simulink model "sliding_mode_controller"  (R2020a)
settings: Solver=ode1  StartTime=0.0  StopTime=50  FixedStep=0.01  RelTol=1e-3
model workspace (MAT data in the model file):
  kd = 0
  kp = 0
libraries: simulink x1, sharedutil x1
settings Model: Creator=Sebas  LastModifiedBy=Sebas
settings SolverCC: ConcurrentTasks=on  ZeroCrossAlgorithm=Adaptive  AlgebraicLoopSolver=LineSearch
settings DebuggingCC: MaskedZcDiagnostic=none  IgnoredZcDiagnostic=none

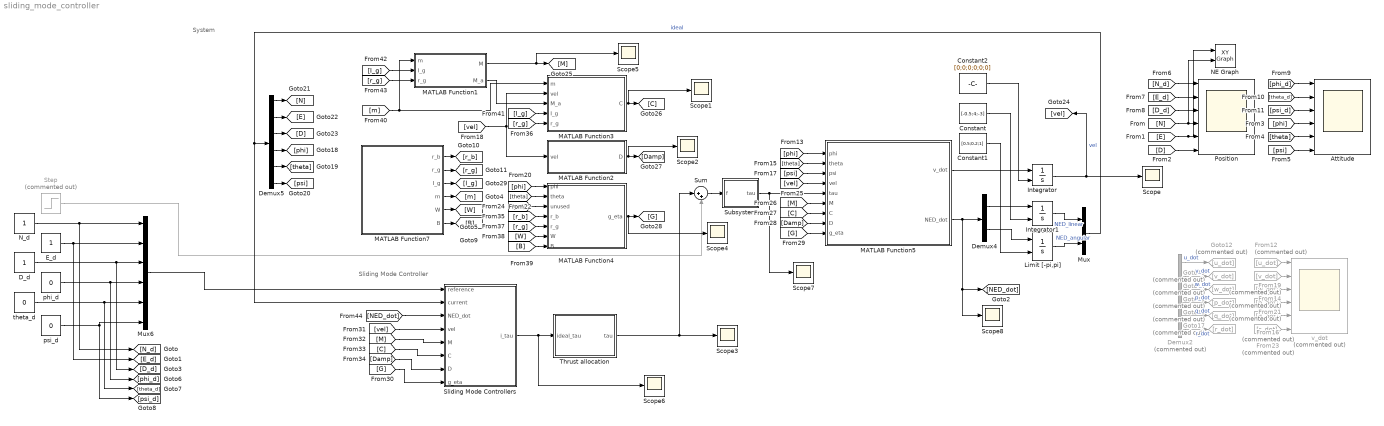
== system sliding_mode_controller ==
  note: System
  note: Sliding Mode Controller
  Attitude : Scope  NumInputPorts=6
  Constant : Constant  Value=[-0.5;4;-3]
  Constant1 : Constant  Value=[0.5;0.2;1]
  Constant2 : Constant  Value=[0;0;0;0;0;0]
  D_d : Constant
  Demux2 : Demux  Commented=on  Outputs=6
  Demux4 : Demux  Outputs=2
  Demux5 : Demux  Outputs=6
  E_d : Constant
  From12 : From  Commented=on  GotoTag=u_dot
  From14 : From  Commented=on  GotoTag=w_dot
  From16 : From  Commented=on  GotoTag=q_dot
  From19 : From  Commented=on  GotoTag=v_dot
  From21 : From  Commented=on  GotoTag=p_dot
  From23 : From  Commented=on  GotoTag=r_dot
  Goto12 : Goto  Commented=on  GotoTag=u_dot
  Goto13 : Goto  Commented=on  GotoTag=v_dot
  Goto14 : Goto  Commented=on  GotoTag=w_dot
  Goto15 : Goto  Commented=on  GotoTag=p_dot
  Goto16 : Goto  Commented=on  GotoTag=q_dot
  Goto17 : Goto  Commented=on  GotoTag=r_dot
  Integrator : Integrator  InitialConditionSource=external
  Integrator1 : Integrator  InitialConditionSource=external
  Limit [-pi,pi] : Integrator  InitialConditionSource=external  WrapState=on
  MATLAB Function1 : MATLAB Function  TreatAsAtomicUnit=on
  MATLAB Function2 : MATLAB Function  TreatAsAtomicUnit=on
  MATLAB Function3 : MATLAB Function  TreatAsAtomicUnit=on
  MATLAB Function4 : MATLAB Function  TreatAsAtomicUnit=on
  MATLAB Function5 : MATLAB Function  TreatAsAtomicUnit=on
  MATLAB Function7 : MATLAB Function  TreatAsAtomicUnit=on
  Mux : Mux  Inputs=2
  Mux6 : Mux  Inputs=6
  NE Graph : simulink/Sinks/XY Graph  xmin=-1  xmax=5  ymin=-1  ymax=2  st=-1
  N_d : Constant
  Position : Scope  NumInputPorts=6
  Scope{,1..8} (9 alike) : Scope
  Sliding Mode Controllers : Subsystem  mask(6 DOF Sliding Mode Controller){surge_k=3, sway_k=3, heave_k=4, roll_k=10, pitch_k=2, yaw_k=5, lambda=1, lambda_roll=5, lambda_pitch=3}
      mask prompts: surge_k "Surge"; sway_k "Sway"; heave_k "Heave"; roll_k "Roll"; pitch_k "Pitch"; yaw_k "Yaw"
      mask help: Implementation of 6 Sliding Mode Controllers for each degree of freedom
      mask DialogControl ParameterGroupVar Prompt: Gains
  Step : Step  Commented=on  Time=20  After=[30;30;30;5;5;5]  SampleTime=0
  Subsystem : Subsystem
  Sum : Sum  Inputs=|++
  Thrust allocation : Subsystem
  phi_d : Constant  Value=0
  psi_d : Constant  Value=0
  theta_d : Constant  Value=0
  v_dot : Scope  Commented=on  NumInputPorts=6
  wires:
  [N_d] -> Position/1
  [E_d] -> Position/2
  [D_d] -> Position/3
  [N] -> Position/4, NE Graph/2
  [D] -> Position/6
  [E] -> Position/5, NE Graph/1
  [phi_d] -> Attitude/1
  [phi] -> Attitude/4
  [psi_d] -> Attitude/3
  [theta] -> Attitude/5
  [psi] -> Attitude/6
  [theta_d] -> Attitude/2
  From12/1 -> v_dot/1
  From19/1 -> v_dot/2
  From14/1 -> v_dot/3
  From21/1 -> v_dot/4
  From16/1 -> v_dot/5
  From23/1 -> v_dot/6
  Demux2/1 -> Goto12/1  "u_dot"
  Demux2/5 -> Goto16/1  "q_dot"
  Demux2/3 -> Goto14/1  "w_dot"
  Demux2/6 -> Goto17/1  "r_dot"
  Demux2/4 -> Goto15/1  "p_dot"
  Demux2/2 -> Goto13/1  "v_dot"
  D_d/1 -> Mux6/3, [D_d]
  theta_d/1 -> Mux6/5, [theta_d]
  phi_d/1 -> Mux6/4, [phi_d]
  E_d/1 -> Mux6/2, [E_d]
  N_d/1 -> Mux6/1, [N_d]
  psi_d/1 -> [psi_d], Mux6/6
  MATLAB Function5/1(v_dot) -> Integrator/1
  MATLAB Function5/2(NED_dot) -> [NED_dot], Scope8/1, Demux4/1
  Demux4/1 -> Integrator1/1
  Demux4/2 -> Limit [-pi,pi]/1
  Limit [-pi,pi]/1 -> Mux/2  "NED_angular"
  Integrator1/1 -> Mux/1  "NED_linear"
  Integrator/1 -> Scope/1, [vel]  "vel"
  Mux6/1 -> Sliding Mode Controllers/1("reference ")
  Sliding Mode Controllers/1(i_tau) -> Scope6/1, Thrust allocation/1(ideal_tau)
  Step/1 -> Sum/2
  Sum/1 -> Subsystem/1(f)
  MATLAB Function1/2(M_a) -> MATLAB Function3/3(M_a)
  Subsystem/1(tau) -> Scope7/1, MATLAB Function5/5(tau)
  Demux5/4 -> [phi]
  Demux5/5 -> [theta]
  Demux5/6 -> [psi]
  [phi] -> MATLAB Function5/1(phi)
  [theta] -> MATLAB Function5/2(theta)
  [psi] -> MATLAB Function5/3(psi)
  Demux5/2 -> [E]
  Demux5/1 -> [N]
  Demux5/3 -> [D]
  [vel] -> MATLAB Function2/1(vel), MATLAB Function3/2(vel)
  [phi] -> MATLAB Function4/1(phi)
  [theta] -> MATLAB Function4/2(theta)
  [psi] -> MATLAB Function4/3(unused)
  [vel] -> MATLAB Function5/4(vel)
  MATLAB Function1/1(M) -> Scope5/1, [M]
  [M] -> MATLAB Function5/6(M)
  MATLAB Function3/1(C) -> Scope1/1, [C]
  [C] -> MATLAB Function5/7(C)
  MATLAB Function2/1(D) -> Scope2/1, [Damp]
  [Damp] -> MATLAB Function5/8(D)
  MATLAB Function4/1(g_eta) -> Scope4/1, [G]
  [G] -> MATLAB Function5/9(g_eta)
  [G] -> Sliding Mode Controllers/8(g_eta)
  Mux/1 -> Sliding Mode Controllers/2(current), Demux5/1  "ideal"
  [vel] -> Sliding Mode Controllers/4(vel)
  [C] -> Sliding Mode Controllers/6(C)
  [Damp] -> Sliding Mode Controllers/7(D)
  [M] -> Sliding Mode Controllers/5(M)
  Constant2/1 -> Integrator/2
  Constant/1 -> Integrator1/2
  Constant1/1 -> Limit [-pi,pi]/2
  MATLAB Function7/2(r_g) -> [r_g]
  MATLAB Function7/1(r_b) -> [r_b]
  MATLAB Function7/3(I_g) -> [I_g]
  MATLAB Function7/4(m) -> [m]
  MATLAB Function7/5(W) -> [W]
  MATLAB Function7/6(B) -> [B]
  [r_b] -> MATLAB Function4/4(r_b)
  [I_g] -> MATLAB Function3/4(I_g)
  [r_g] -> MATLAB Function4/5(r_g)
  [W] -> MATLAB Function4/6(W)
  [B] -> MATLAB Function4/7(B)
  [m] -> MATLAB Function3/1(m), MATLAB Function1/1(m)
  [r_g] -> MATLAB Function3/5(r_g)
  [I_g] -> MATLAB Function1/2(I_g)
  [r_g] -> MATLAB Function1/3(r_g)
  Thrust allocation/1(tau) -> Scope3/1, Sum/1
  [NED_dot] -> Sliding Mode Controllers/3(NED_dot)

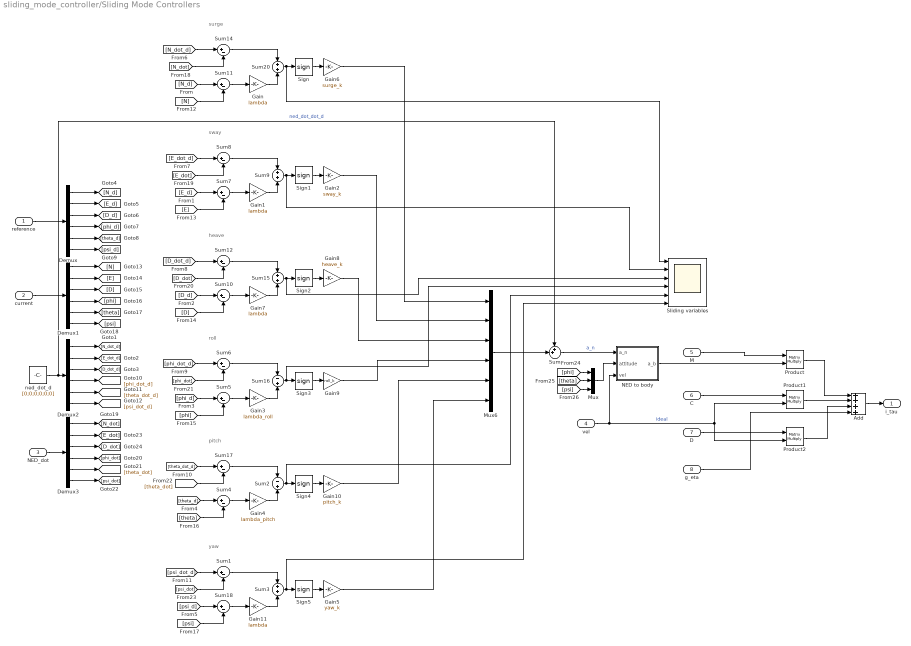
== system sliding_mode_controller/Sliding Mode Controllers ==
  note: surge
  note: sway
  note: heave
  note: roll
  note: pitch
  note: yaw
  "reference " : Inport
  current : Inport  Port=2
  NED_dot : Inport  Port=3
  vel : Inport  Port=4
  M : Inport  Port=5
  C : Inport  Port=6
  D : Inport  Port=7
  g_eta : Inport  Port=8
  Add : Sum  Inputs=4
  Demux{,1..3} (4 alike) : Demux  Outputs=6
  Gain{,1,7,11} (4 alike) : Gain  Gain=lambda
  Gain10 : Gain  Gain=pitch_k
  Gain2 : Gain  Gain=sway_k
  Gain3 : Gain  Gain=lambda_roll
  Gain4 : Gain  Gain=lambda_pitch
  Gain5 : Gain  Gain=yaw_k
  Gain6 : Gain  Gain=surge_k
  Gain8 : Gain  Gain=heave_k
  Gain9 : Gain  Gain=roll_k
  Mux : Mux  Inputs=3
  Mux6 : Mux  Inputs=6
  NED to body : Subsystem
  Product : Product  Multiplication=Matrix(*)
  Product1 : Product  Multiplication=Matrix(*)
  Product2 : Product  Multiplication=Matrix(*)
  Sign{,1..5} (6 alike) : Signum  ZeroCross=off
  Sliding variables : Scope  NumInputPorts=6
  Sum : Sum  Inputs=++|
  Sum{1,4..8,10..12,14,17..18} (12 alike) : Sum  Inputs=|+-
  Sum{3,9,15,20} (4 alike) : Sum
  Sum16 : Sum  Inputs=-+
  Sum2 : Sum  Inputs=-+
  ned_dot_d : Constant  Value=[0;0;0;0;0;0]
  i_tau : Outport
  wires:
  Gain8/1 -> Mux6/3
  Gain10/1 -> Mux6/5
  Gain9/1 -> Mux6/4
  Gain5/1 -> Mux6/6
  Gain6/1 -> Mux6/1
  Gain2/1 -> Mux6/2
  Sum14/1 -> Sum20/1
  Sum11/1 -> Gain/1
  current/1 -> Demux1/1
  Demux1/1 -> [N]
  "reference "/1 -> Demux/1
  Demux/1 -> [N_d]
  Demux1/2 -> [E]
  Demux/3 -> [D_d]
  Demux1/3 -> [D]
  Demux/4 -> [phi_d]
  Demux1/4 -> [phi]
  Demux/5 -> [theta_d]
  Demux1/5 -> [theta]
  Demux/6 -> [psi_d]
  Demux1/6 -> [psi]
  Add/1 -> i_tau/1
  Product1/1 -> Add/2
  Demux2/1 -> [N_dot_d]
  Demux3/1 -> [N_dot]
  Demux2/2 -> [E_dot_d]
  Demux3/2 -> [E_dot]
  Demux2/3 -> [D_dot_d]
  Demux3/3 -> [D_dot]
  Demux2/4 -> [phi_dot_d]
  Demux3/4 -> [phi_dot]
  Demux2/5 -> [theta_dot_d]
  Demux3/5 -> [theta_dot]
  Demux3/6 -> [psi_dot]
  Demux2/6 -> [psi_dot_d]
  [N_d] -> Sum11/1
  Demux/2 -> [E_d]
  [phi_d] -> Sum5/1
  [psi_d] -> Sum18/1
  [N_dot_d] -> Sum14/1
  [phi_dot_d] -> Sum6/1
  [psi_dot_d] -> Sum1/1
  [N] -> Sum11/2
  [phi] -> Sum5/2
  [theta] -> Sum4/2
  [psi] -> Sum18/2
  [N_dot] -> Sum14/2
  Gain/1 -> Sum20/2
  Sum20/1 -> Sliding variables/1, Sign/1
  Sign/1 -> Gain6/1
  Sign1/1 -> Gain2/1
  Sum9/1 -> Sliding variables/2, Sign1/1
  Gain1/1 -> Sum9/2
  [E_dot] -> Sum8/2
  [E] -> Sum7/2
  Sum7/1 -> Gain1/1
  Sum8/1 -> Sum9/1
  Sum12/1 -> Sum15/1
  Sum10/1 -> Gain7/1
  Gain7/1 -> Sum15/2
  Sum15/1 -> Sliding variables/3, Sign2/1
  Sign2/1 -> Gain8/1
  Sign3/1 -> Gain9/1
  Sum16/1 -> Sliding variables/4, Sign3/1
  Gain3/1 -> Sum16/2
  Sum5/1 -> Gain3/1
  Sum6/1 -> Sum16/1
  [E_dot_d] -> Sum8/1
  [E_d] -> Sum7/1
  [D_dot_d] -> Sum12/1
  [D_dot] -> Sum12/2
  [D_d] -> Sum10/1
  [D] -> Sum10/2
  [phi_dot] -> Sum6/2
  Sum17/1 -> Sum2/1
  Sum4/1 -> Gain4/1
  Gain4/1 -> Sum2/2
  Sum2/1 -> Sliding variables/5, Sign4/1
  Sign4/1 -> Gain10/1
  [theta_dot_d] -> Sum17/1
  [theta_dot] -> Sum17/2
  [theta_d] -> Sum4/1
  Sign5/1 -> Gain5/1
  Sum3/1 -> Sliding variables/6, Sign5/1
  Gain11/1 -> Sum3/2
  Sum18/1 -> Gain11/1
  Sum1/1 -> Sum3/1
  [psi_dot] -> Sum1/2
  ned_dot_d/1 -> Sum/1, Demux2/1  "ned_dot_dot_d"
  Mux6/1 -> Sum/2
  Product/1 -> Add/1
  M/1 -> Product/1
  C/1 -> Product1/1
  D/1 -> Product2/1
  vel/1 -> NED to body/3(vel), Product2/2, Product1/2  "ideal"
  Product2/1 -> Add/3
  g_eta/1 -> Add/4
  NED_dot/1 -> Demux3/1
  Sum/1 -> NED to body/1(a_n)  "a_n"
  [phi] -> Mux/1
  [theta] -> Mux/2
  [psi] -> Mux/3
  Mux/1 -> NED to body/2(attitude)
  NED to body/1(a_b) -> Product/2

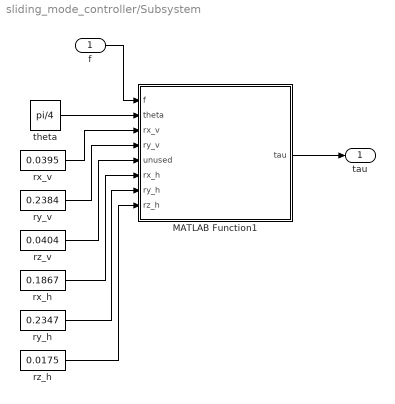
== system sliding_mode_controller/Subsystem ==
  f : Inport
  MATLAB Function1 : MATLAB Function  TreatAsAtomicUnit=on
  rx_h : Constant  Value=0.1867
  rx_v : Constant  Value=0.0395
  ry_h : Constant  Value=0.2347
  ry_v : Constant  Value=0.2384
  rz_h : Constant  Value=0.0175
  rz_v : Constant  Value=0.0404
  theta : Constant  Value=pi/4
  tau : Outport
  wires:
  rz_v/1 -> MATLAB Function1/5(unused)
  ry_h/1 -> MATLAB Function1/7(ry_h)
  f/1 -> MATLAB Function1/1(f)
  MATLAB Function1/1(tau) -> tau/1
  rx_h/1 -> MATLAB Function1/6(rx_h)
  theta/1 -> MATLAB Function1/2(theta)
  rx_v/1 -> MATLAB Function1/3(rx_v)
  rz_h/1 -> MATLAB Function1/8(rz_h)
  ry_v/1 -> MATLAB Function1/4(ry_v)

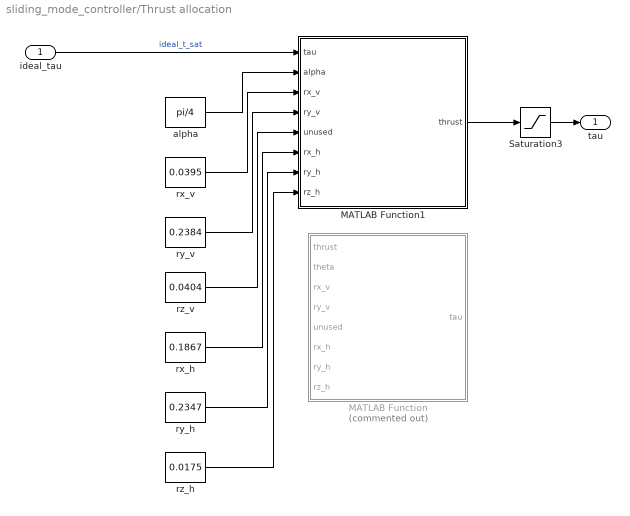
== system sliding_mode_controller/Thrust allocation ==
  ideal_tau : Inport
  MATLAB Function : MATLAB Function  Commented=on  TreatAsAtomicUnit=on
  MATLAB Function1 : MATLAB Function  TreatAsAtomicUnit=on
  Saturation3 : Saturate  UpperLimit=35  LowerLimit=-35
  alpha : Constant  Value=pi/4
  rx_h : Constant  Value=0.1867
  rx_v : Constant  Value=0.0395
  ry_h : Constant  Value=0.2347
  ry_v : Constant  Value=0.2384
  rz_h : Constant  Value=0.0175
  rz_v : Constant  Value=0.0404
  tau : Outport
  wires:
  ideal_tau/1 -> MATLAB Function1/1(tau)  "ideal_t_sat"
  MATLAB Function1/1(thrust) -> Saturation3/1
  Saturation3/1 -> tau/1
  rx_v/1 -> MATLAB Function1/3(rx_v)
  alpha/1 -> MATLAB Function1/2(alpha)
  rx_h/1 -> MATLAB Function1/6(rx_h)
  ry_h/1 -> MATLAB Function1/7(ry_h)
  rz_h/1 -> MATLAB Function1/8(rz_h)
  ry_v/1 -> MATLAB Function1/4(ry_v)
  rz_v/1 -> MATLAB Function1/5(unused)

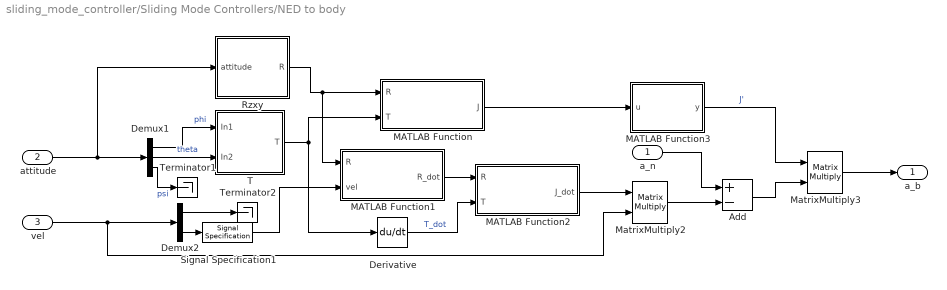
== system sliding_mode_controller/Sliding Mode Controllers/NED to body ==
  a_n : Inport
  attitude : Inport  Port=2
  vel : Inport  Port=3
  Add : Sum  Inputs=+-
  Demux1 : Demux  Outputs=3
  Demux2 : Demux  Outputs=2
  Derivative : Derivative
  MATLAB Function : MATLAB Function  TreatAsAtomicUnit=on
  MATLAB Function1 : MATLAB Function  TreatAsAtomicUnit=on
  MATLAB Function2 : MATLAB Function  TreatAsAtomicUnit=on
  MATLAB Function3 : MATLAB Function  TreatAsAtomicUnit=on
  MatrixMultiply2 : Product  Multiplication=Matrix(*)
  MatrixMultiply3 : Product  Multiplication=Matrix(*)
  Rzxy : Subsystem
  Signal Specification1 : SignalSpecification  Dimensions=3
  T : Subsystem
  Terminator1 : Terminator
  Terminator2 : Terminator
  a_b : Outport
  wires:
  a_n/1 -> Add/1
  attitude/1 -> Demux1/1, Rzxy/1(attitude)
  Demux1/1 -> T/1(In1)  "phi"
  Demux1/2 -> T/2(In2)  "theta"
  MATLAB Function/1(J) -> MATLAB Function3/1(u)
  Demux1/3 -> Terminator1/1  "psi"
  Rzxy/1(R) -> MATLAB Function1/1(R), MATLAB Function/1(R)
  T/1(T) -> Derivative/1, MATLAB Function/2(T)
  MATLAB Function1/1(R_dot) -> MATLAB Function2/1(R)
  Derivative/1 -> MATLAB Function2/2(T)  "T_dot"
  Demux2/1 -> Terminator2/1
  MatrixMultiply2/1 -> Add/2
  Add/1 -> MatrixMultiply3/2
  MatrixMultiply3/1 -> a_b/1
  Demux2/2 -> Signal Specification1/1
  MATLAB Function3/1(y) -> MatrixMultiply3/1  "J'"
  vel/1 -> Demux2/1, MatrixMultiply2/2
  Signal Specification1/1 -> MATLAB Function1/2(vel)
  MATLAB Function2/1(J_dot) -> MatrixMultiply2/1

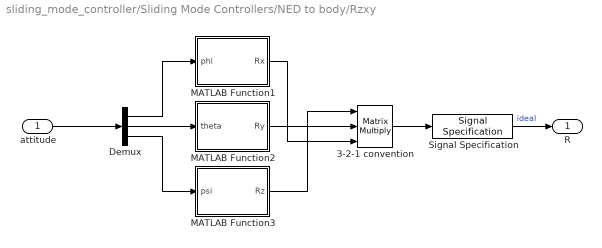
== system sliding_mode_controller/Sliding Mode Controllers/NED to body/Rzxy ==
  attitude : Inport
  3-2-1 convention : Product  Inputs=3  Multiplication=Matrix(*)
  Demux : Demux  Outputs=3
  MATLAB Function1 : MATLAB Function  TreatAsAtomicUnit=on
  MATLAB Function2 : MATLAB Function  TreatAsAtomicUnit=on
  MATLAB Function3 : MATLAB Function  TreatAsAtomicUnit=on
  Signal Specification : SignalSpecification  Dimensions=[3,3]
  R : Outport
  wires:
  Demux/1 -> MATLAB Function1/1(phi)
  MATLAB Function3/1(Rz) -> 3-2-1 convention/1
  MATLAB Function2/1(Ry) -> 3-2-1 convention/2
  Demux/3 -> MATLAB Function3/1(psi)
  MATLAB Function1/1(Rx) -> 3-2-1 convention/3
  3-2-1 convention/1 -> Signal Specification/1
  attitude/1 -> Demux/1
  Demux/2 -> MATLAB Function2/1(theta)
  Signal Specification/1 -> R/1  "ideal"

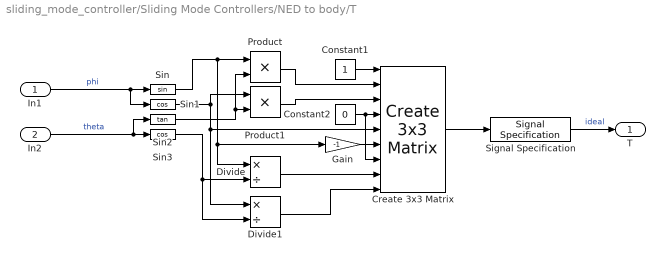
== system sliding_mode_controller/Sliding Mode Controllers/NED to body/T ==
  In1 : Inport
  In2 : Inport  Port=2
  Constant1 : Constant
  Constant2 : Constant  Value=0
  Create 3x3 Matrix : sharedutil/Create 3x3 Matrix  aMode=aMode
      settings: SourceProductBaseCode=AE,PW,MT,VE,VP
  Divide : Product  Inputs=*/
  Divide1 : Product  Inputs=*/
  Gain : Gain  Gain=-1
  Product : Product
  Product1 : Product
  Signal Specification : SignalSpecification  Dimensions=[3,3]
  Sin : Trigonometry
  Sin1 : Trigonometry  Operator=cos
  Sin2 : Trigonometry  Operator=tan
  Sin3 : Trigonometry  Operator=cos
  T : Outport
  wires:
  Constant2/1 -> Create 3x3 Matrix/7, Create 3x3 Matrix/4
  Gain/1 -> Create 3x3 Matrix/6
  Divide1/1 -> Create 3x3 Matrix/9
  Product/1 -> Create 3x3 Matrix/2
  Sin1/1 -> Divide1/1, Create 3x3 Matrix/5, Product1/1
  In1/1 -> Sin1/1, Sin/1  "phi"
  Sin2/1 -> Product/2, Product1/2
  Divide/1 -> Create 3x3 Matrix/8
  Product1/1 -> Create 3x3 Matrix/3
  Sin3/1 -> Divide1/2, Divide/2
  In2/1 -> Sin2/1, Sin3/1  "theta"
  Sin/1 -> Gain/1, Divide/1, Product/1
  Constant1/1 -> Create 3x3 Matrix/1
  Create 3x3 Matrix/1 -> Signal Specification/1
  Signal Specification/1 -> T/1  "ideal"

== matlab function sliding_mode_controller/Sliding Mode Controllers/NED to body/MATLAB Function2 ==
  data: R input; J_dot output; T input
function J_dot = diff_transform_matrix(R,T)
J_dot = [R          zeros(3);
         zeros(3)    T];

== matlab function sliding_mode_controller/Sliding Mode Controllers/NED to body/MATLAB Function3 ==
  data: u input; y output
function y = fcn(u)
y = inv(u);

== matlab function sliding_mode_controller/Thrust allocation/MATLAB Function1 ==
  data: tau input; thrust output; alpha input; rx_v input; ry_v input; unused input; rx_h input; ry_h input; rz_h input
function thrust = thrust_allocation(tau, alpha, rx_v, ry_v, ~, rx_h, ry_h, rz_h)
% Mapping matrix
T = [cos(alpha) cos(alpha) -cos(alpha) -cos(alpha) 0 0;
     -sin(alpha) sin(alpha) -sin(alpha) sin(alpha) 0 0;
     0 0 0 0 -1 -1;
     -sin(alpha)*rz_h sin(alpha)*rz_h -sin(alpha)*rz_h sin(alpha)*rz_h -ry_v ry_v;
     -cos(alpha)*rz_h -cos(alpha)*rz_h cos(alpha)*rz_h cos(alpha)*rz_h -rx_v rx_v;
     -(rx_h*sin(alpha)+ry_h*cos(alpha)) (rx_h*sin(alpha)+ry_h*cos(alpha)) (rx_h*sin(alpha)+ry_h*cos(alpha)) -(rx_h*sin(alpha)+ry_h*cos(alpha)) 0 0
    ];
% Control input with Moore–Penrose pseudo-inverse
t = pinv(T)*tau;
thrust = t;

== matlab function sliding_mode_controller/MATLAB Function2 ==
  data: vel input; D output
function D = Damping(vel)
% Linear damping coefficients
X_u = -0.3431;
Y_v = 0.0518;
Z_w = -0.5841;
K_p = 0.0064;
M_q = 0.04;
N_r = -0.1063;

% Cuadratic damping coefficients
X_uu = -111.7397;
Y_vv = -44.4058;
Z_ww = -157.1951;
K_pp = -0.4634;
M_qq = -0.2902;
N_rr = -2.2897;

% Linear damping matrix
D_lin = -diag([X_u Y_v Z_w K_p M_q N_r]);

% Cuadratic Damping matrix
D_cuad = -diag([X_uu*abs(vel(1)) Y_vv*abs(vel(2)) Z_ww*abs(vel(3)) ...
               K_pp*abs(vel(4)) M_qq*abs(vel(5)) N_rr*abs(vel(6))]);

%Damping matrix
D = D_lin + D_cuad;

== matlab function sliding_mode_controller/MATLAB Function3 ==
  data: m input; vel input; C output; M_a input; I_g input; r_g input
function C = Coriolis(m,vel,M_a,I_g,r_g)
% Skew symmetric matrix
S = @(s) [0    -s(3) s(2);
          s(3) 0     -s(1);
          -s(2) s(1)  0    ];  

% Rigid-body Coriolis-centripetal Matrix
C_rb = [ zeros(3)             -m*S(vel(1:3))-m*S(vel(4:6))*S(r_g);
        -m*S(vel(1:3))+m*S(r_g)*S(vel(4:6))            -S(I_g*vel(4:6))];

% Coreolis added mass matrix 
C_a = [ 0 0 0   0 -M_a(3,3)*vel(3) M_a(2,2)*vel(2) ;
        0 0 0   M_a(3,3)*vel(3) 0 -M_a(1,1)*vel(1) ;
        0 0 0  -M_a(2,2)*vel(2) M_a(1,1)*vel(1) 0  ;
        0 -M_a(3,3)*vel(3) M_a(2,2)*vel(2)  0 -M_a(6,6)*vel(6) M_a(5,5)*vel(5) ;
        M_a(3,3)*vel(3) 0 -M_a(1,1)*vel(1)  M_a(6,6)*vel(6) 0 -M_a(4,4)*vel(4) ;
       -M_a(2,2)*vel(2) M_a(1,1)*vel(1) 0   -M_a(5,5)*vel(5) M_a(4,4)*vel(4) 0  ];

% Coreolis matrix
C = C_rb + C_a;

== matlab function sliding_mode_controller/MATLAB Function4 ==
  data: phi input; g_eta output; theta input; unused input; r_b input; r_g input; W input; B input
function g_eta = Restore(phi,theta,~,r_b,r_g,W,B)
% Restoring forces
g_eta = [ (W-B)*sin(theta);
          -(W-B)*cos(theta)*sin(phi);
          -(W-B)*cos(theta)*cos(phi);
          -(r_g(2)*W-r_b(2)*B)*cos(theta)*cos(phi) + (r_g(3)*W-r_b(3)*B)*cos(theta)*sin(phi);
           (r_g(3)*W-r_b(3)*B)*sin(theta)             + (r_g(1)*W-r_b(1)*B)*cos(theta)*cos(phi)
          -(r_g(1)*W-r_b(1)*B)*cos(theta)*sin(phi) - (r_g(2)*W-r_b(2)*B)*sin(theta)          ];

== matlab function sliding_mode_controller/MATLAB Function5 ==
  data: phi input; theta input; psi input; vel input; tau input; M input; C input; D input; v_dot output; g_eta input; NED_dot output
function [v_dot, NED_dot]= Forward_dynamics(phi,theta,psi,vel,tau,M,C,D,g_eta)
f = M\(-(C*vel)-(D*vel)-g_eta);
g = inv(M);

NED_dot = [ % Linear velocities in NED / For a zxy rotation sequence
            [vel(1)*cos(psi)*cos(theta) + vel(2)*[cos(psi)*sin(theta)*sin(phi)... 
             - sin(psi)*cos(phi)] + vel(3)*[sin(psi)*sin(phi)... 
             + cos(psi)*cos(phi)*sin(theta)]];
            [vel(1)*sin(psi)*cos(theta) + vel(2)*[cos(psi)*cos(phi)... 
             + sin(phi)*sin(theta)*sin(psi)]+ vel(3)*[sin(theta)*sin(psi)*cos(phi)... 
             - cos(psi)*sin(phi)]];
            [-vel(1)*sin(theta) + vel(2)*cos(theta)*sin(phi) + vel(3)*cos(theta)*cos(phi)];
            %Angular velocities in NED
            [vel(4) + vel(5)*sin(phi)*tan(theta) + vel(6)*cos(phi)*tan(theta)];
            [vel(5)*cos(phi) - vel(6)*sin(phi)];
            [vel(5)*(sin(phi)/cos(theta)) + vel(6)*(cos(phi)/cos(theta))];
           ];

v_dot = f + g*tau;

== matlab function sliding_mode_controller/MATLAB Function7 ==
  data: r_b output; r_g output; I_g output; m output; W output; B output
function [r_b,r_g,I_g,m,W,B] = System_parameters()
r_g = [0 0 0].';    % Distance from origin to center of mass
r_b = [0 0 -0.10726].';    % Distance from origin to center of buoyancy
I_g = [0.900121387  -0.000186482 0.0072251;
       -0.000186482 1.754494427  0.020319615;
       0.0072251    0.020319615  1.43389     ]; % Rigid-body inertia matrix
m = 24;
vol = 0.02306187;
W = m*9.81;
B = W*1.005; %1000*9.81*vol;

== matlab function sliding_mode_controller/Sliding Mode Controllers/NED to body/Rzxy/MATLAB Function1 ==
  data: phi input; Rx output
function Rx = Rx(phi)
Rx = [ 1 0 0;
       0 cos(phi) -sin(phi);
       0 sin(phi) cos(phi); ];

== matlab function sliding_mode_controller/MATLAB Function1 ==
  data: m input; M output; M_a output; I_g input; r_g input
function [M,M_a] = Mass_Matrix(m,I_g,r_g)
% Skew symmetric matrix
S = @(s) [0    -s(3) s(2);
          s(3) 0     -s(1);
          -s(2) s(1)  0    ];  

% Rigid-Body Inertia Matrix
M_rb = [ m*eye(3)    -m*S(r_g);
         m*S(r_g)         I_g ];

% Added mass matrix
M_a = diag([16.8374 20.2748 35.3180 0.2165 0.6869 0.6157]);

% Mass matrix
M = M_rb + M_a;

== matlab function sliding_mode_controller/Thrust allocation/MATLAB Function ==
  data: thrust input; tau output; theta input; rx_v input; ry_v input; unused input; rx_h input; ry_h input; rz_h input
function tau = thrust_conversion(thrust, theta, rx_v, ry_v, ~, rx_h, ry_h, rz_h)
% Errores numericos. El input esta saturado a [100,-100], y estas salidas
% dan valores muchisimo mayores a 35 N c/u
tau = [0 0 0 0 0 0].';
% For surge
s_val = thrust(1)/cos(theta)/4;
tau(1) = tau(1)+s_val;
tau(2) = tau(2)+s_val;
tau(3) = tau(3)-s_val;
tau(4) = tau(4)-s_val;

% For sway
sw_val = thrust(2)/sin(theta)/4;
tau(1) = tau(1)-sw_val;
tau(2) = tau(2)+sw_val;
tau(3) = tau(3)-sw_val;
tau(4) = tau(4)+sw_val;

% For heave
tau(5) = tau(5)+(-thrust(3)/2);
tau(6) = tau(6)+(-thrust(3)/2);

% For yaw
y_val = thrust(6)/(rx_h*sin(theta)+ry_h*cos(theta))/4;
tau(1) = tau(1)-y_val;
tau(2) = tau(2)+y_val;
tau(3) = tau(3)+y_val;
tau(4) = tau(4)-y_val;

% K and M come as zero
% For K
if  thrust(4)~= 0
    %disp("K")
    k_val = (thrust(4)-(-tau(1)+tau(2)-tau(3)+tau(4))*sin(theta)*rz_h)/(2*ry_v);
    tau(5) = tau(5)-k_val;
    tau(6) = tau(6)+k_val;
end

% For M
if thrust(5) ~= 0
    %disp("M")
    M_val = (thrust(5)-(-tau(1)-tau(2)+tau(3)+tau(4))*cos(theta)*rz_h)/(2*rx_v);
    tau(5) = tau(5)-M_val;
    tau(6) = tau(6)+M_val;
end
disp(tau)

== matlab function sliding_mode_controller/Sliding Mode Controllers/NED to body/MATLAB Function ==
  data: R input; J output; T input
function J = transform_matrix(R,T)
J= [R          zeros(3);
     zeros(3)    T];

== matlab function sliding_mode_controller/Subsystem/MATLAB Function1 ==
  data: tau output; f input; theta input; rx_v input; ry_v input; unused input; rx_h input; ry_h input; rz_h input
function tau = tau_conversion(f, theta, rx_v, ry_v, ~, rx_h, ry_h, rz_h)
tau = [0 0 0 0 0 0].';
tau(1) = (f(1)+f(2)-f(3)-f(4))*cos(theta);
tau(2) = (-f(1)+f(2)-f(3)+f(4))*sin(theta);
tau(3) = -(f(5)+f(6));
tau(4) = (f(6)-f(5))*ry_v + (-f(1)+f(2)-f(3)+f(4))*sin(theta)*rz_h;
tau(5) = (f(6)-f(5))*rx_v + (-f(1)-f(2)+f(3)+f(4))*cos(theta)*rz_h;
tau(6) = (-f(1)+f(2)+f(3)-f(4))*(rx_h*sin(theta)+ry_h*cos(theta));

== matlab function sliding_mode_controller/Sliding Mode Controllers/NED to body/Rzxy/MATLAB Function2 ==
  data: theta input; Ry output
function Ry = Ry(theta)
Ry = [ cos(theta) 0 sin(theta);
       0          1     0 ;
       -sin(theta) 0 cos(theta); ];

== matlab function sliding_mode_controller/Sliding Mode Controllers/NED to body/Rzxy/MATLAB Function3 ==
  data: psi input; Rz output
function Rz = Rz(psi)
Rz = [ cos(psi) -sin(psi) 0;
       sin(psi) cos(psi)  0;
       0        0         1];

== matlab function sliding_mode_controller/Sliding Mode Controllers/NED to body/MATLAB Function1 ==
  data: R input; vel input; R_dot output
function R_dot = Diff_Rot_matrix(R,vel)
% Skew symmetric matrix
a = [0    -vel(3) vel(2);
     vel(3) 0     -vel(1);
     -vel(2) vel(1)  0    ];
R_dot = R*a;
